simulink model "chap7_2sim_matlabfunction"  (Simulink 8.4)
settings: Solver=ode1  StartTime=0.0  StopTime=10  FixedStep=0.001  RelTol=1e-3
values from neighbouring files (symbols this model uses):
  input = [0 0.00314157198278 0.00628301994168 0.0094242198577 0.0125650477217 0.0157053795391 0.018845091335 0.0219840591589 0.0251221590899 0.028259267241 0.0313952597647 0.0345300128572 ... (10001 elements, 10001x1)]    [input.mat]
  PlantADen = [1 PlantAPara.a1 PlantAPara.a0]    [main.m]
  PlantANum = [PlantAPara.b1 PlantAPara.b0]    [main.m]
  s = u(1)    [chap7_2ctrl.m]    (also in fsmcctrl.m)
  Ts = 0.001    [main.m]
libraries: simulink x5, fod x3
settings Model: Creator=Administrator  LastModifiedBy=Administrator  ExtModeTrigMode=oneshot  ExtModeArmWhenConnect=off
settings DataIOCC: LimitDataPoints=off  SignalLoggingName=sigsOut
settings OptimizationCC: BooleanDataType=off  ExpressionDepthLimit=128
settings DebuggingCC: SaveWithParameterizedLinksMsg=none  SignalResolutionControl=TryResolveAllWithWarning  SolverPrmCheckMsg=none  MultiTaskDSMMsg=warning  MultiTaskCondExecSysMsg=none  FcnCallInpInsideContextMsg=EnableAllAsError  StateNameClashWarn=none
settings HardwareCC: TargetLongLongMode=on  TargetIntDivRoundTo=Zero  TargetEndianess=LittleEndian  TargetHWDeviceType=MATLAB Host  ProdEqTarget=off
settings RTWCC: IncludeERTFirstTime=on

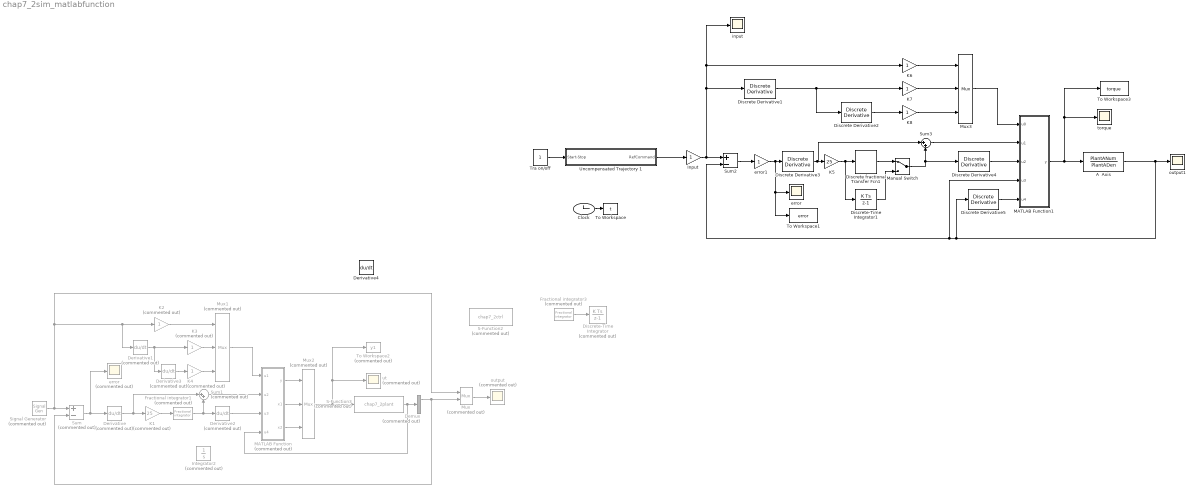
== system chap7_2sim_matlabfunction ==
  A  Axis : DiscreteTransferFcn  Numerator=PlantANum  Denominator=PlantADen  SampleTime=Ts
  Clock : Clock
  Demux : Demux  Commented=on  Outputs=2
  Derivative{,1..3} (4 alike) : Derivative  Commented=on
  Derivative4 : Derivative
  Discrete Derivative{1..5} (5 alike) : simulink/Discrete/Discrete Derivative  gainval=1.0  ICPrevScaledInput=0.0  InputProcessing=Inherited  OutMin=[]  OutMax=[]  OutDataType=fixdt(1, 16)  OutScaling=2^-10  DoSatur=off
  Discrete fractional Transfer Fcn1 : fod/Discrete fractional Transfer Fcn  zeroPoly=1  polePoly=s^0.9  freqRange=[0.001, 1000]  approxNum=5  useRef=off  dscrMethod=Matched  wc=0  ts=0.001
  Discrete-Time Integrator : DiscreteIntegrator  Commented=on  InitialConditionSetting=State (most efficient)
  Discrete-Time Integrator1 : DiscreteIntegrator  InitialConditionSetting=State (most efficient)  SampleTime=0.001
  Fractional integrator1 : fod/Fractional integrator  Commented=on  gam=0.7  ww=[0.001; 1000]  n=3  nFod=off
  Fractional integrator3 : fod/Fractional integrator  Commented=on  gam=0.9  ww=[0.001; 1000]  n=3  nFod=off
  Input : Gain  SampleTime=0.001
  Integrator2 : Integrator  Commented=on
  K1 : Gain  Commented=on  Gain=25
  K2 : Gain  Commented=on
  K3 : Gain  Commented=on
  K4 : Gain  Commented=on
  K5 : Gain  Gain=25  SampleTime=0.001
  K6 : Gain
  K7 : Gain
  K8 : Gain
  MATLAB Function : MATLAB Function  Commented=on  TreatAsAtomicUnit=on
  MATLAB Function1 : MATLAB Function  TreatAsAtomicUnit=on
  Manual Switch : ManualSwitch
  Mux : Mux  Commented=on  Inputs=2
  Mux1 : Mux  Commented=on  Inputs=3
  Mux2 : Mux  Commented=on  Inputs=3
  Mux3 : Mux  Inputs=3
  S-Function2 : S-Function  Commented=on  FunctionName=chap7_2ctrl  EnableBusSupport=off
  S-Function3 : S-Function  Commented=on  FunctionName=chap7_2plant  EnableBusSupport=off
  Signal Generator : SignalGenerator  Commented=on
  Sum : Sum  Commented=on  Inputs=+-  SaturateOnIntegerOverflow=on  InputSameDT=on  OutDataTypeStr=Inherit: Same as first input
  Sum1 : Sum  Commented=on  Inputs=|++
  Sum2 : Sum  Inputs=+-  SampleTime=0.001  SaturateOnIntegerOverflow=on  InputSameDT=on  OutDataTypeStr=Inherit: Same as first input
  Sum3 : Sum  Inputs=|++  SampleTime=0.001
  To Workspace : ToWorkspace  VariableName=t  SampleTime=-1
  To Workspace1 : ToWorkspace  VariableName=error  SampleTime=-1
  To Workspace2 : ToWorkspace  Commented=on  VariableName=y1  SampleTime=-1
  To Workspace3 : ToWorkspace  VariableName=torque  SampleTime=-1
  "Tra on/off " : Constant  SampleTime=0.001
  Uncompensated Trajectory 1 : Subsystem
  error : Scope  Commented=on
      settings: SaveName=ScopeData2
  "error " : Scope
      settings: SaveName=ScopeData5
  error1 : Gain  SampleTime=0.001
  "input " : Scope
      settings: SaveName=ScopeData4
  output : Scope  Commented=on
  output1 : Scope
  "torque " : Scope
      settings: SaveName=ScopeData6
  ut : Scope  Commented=on
      settings: SaveName=ScopeData3
  wires:
  Clock/1 -> To Workspace/1
  Mux2/1 -> To Workspace2/1, ut/1, S-Function3/1
  Mux/1 -> output/1
  Sum/1 -> Derivative/1, error/1
  Signal Generator/1 -> K2/1, Derivative1/1, Mux/1, Sum/1
  Demux/1 -> Sum/2, Mux/2
  Derivative/1 -> Sum1/1, K1/1
  Sum1/1 -> MATLAB Function/2(u2)
  K1/1 -> Fractional integrator1/1
  Fractional integrator1/1 -> Derivative2/1, Sum1/2
  Derivative2/1 -> MATLAB Function/3(u3)
  Derivative1/1 -> K3/1, Derivative3/1
  Derivative3/1 -> K4/1
  K2/1 -> Mux1/1
  K3/1 -> Mux1/2
  K4/1 -> Mux1/3
  Mux1/1 -> MATLAB Function/1(u1)
  S-Function3/1 -> MATLAB Function/4(u4), Demux/1
  MATLAB Function/1(y) -> Mux2/1
  MATLAB Function/2(x1) -> Mux2/2
  MATLAB Function/3(x2) -> Mux2/3
  Sum2/1 -> error1/1
  Discrete Derivative3/1 -> Sum3/1, K5/1
  Sum3/1 -> MATLAB Function1/2(u1)
  K5/1 -> Discrete-Time Integrator1/1, Discrete fractional Transfer Fcn1/1
  Discrete fractional Transfer Fcn1/1 -> Manual Switch/1
  Discrete Derivative4/1 -> MATLAB Function1/3(u2)
  A  Axis/1 -> Discrete Derivative5/1, Sum2/2, MATLAB Function1/4(u3), output1/1
  Discrete Derivative5/1 -> MATLAB Function1/5(u4)
  "Tra on/off "/1 -> Uncompensated Trajectory 1/1(Start-Stop)
  error1/1 -> To Workspace1/1, "error "/1, Discrete Derivative3/1
  Discrete Derivative1/1 -> Discrete Derivative2/1, K7/1
  Discrete Derivative2/1 -> K8/1
  K6/1 -> Mux3/1
  K7/1 -> Mux3/2
  K8/1 -> Mux3/3
  Mux3/1 -> MATLAB Function1/1(u0)
  Input/1 -> Discrete Derivative1/1, "input "/1, K6/1, Sum2/1
  MATLAB Function1/1(y) -> To Workspace3/1, "torque "/1, A  Axis/1
  Fractional integrator3/1 -> Discrete-Time Integrator/1
  Uncompensated Trajectory 1/1(RefCommand) -> Input/1
  Discrete-Time Integrator1/1 -> Manual Switch/2
  Manual Switch/1 -> Discrete Derivative4/1, Sum3/2

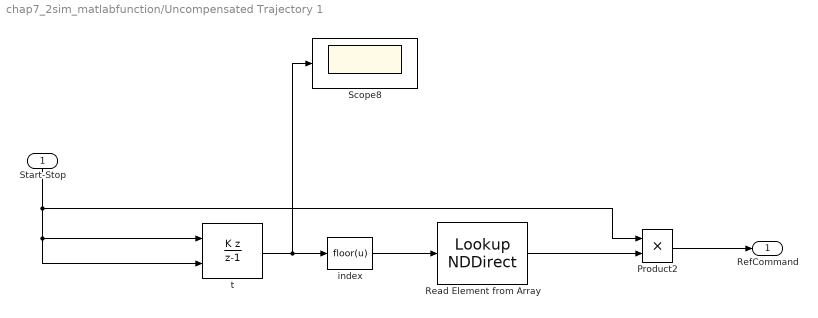
== system chap7_2sim_matlabfunction/Uncompensated Trajectory 1 ==
  Start-Stop : Inport
  Product2 : Product  RndMeth=Zero
  Read Element from Array : LookupNDDirect  NumberOfTableDimensions=1  Table=input
  Scope8 : Scope
      settings: YMin=-50  YMax=250  SaveName=ScopeData9
  index : Fcn  Expr=floor(u)
  t : DiscreteIntegrator  IntegratorMethod=Accumulation: Backward Euler  ExternalReset=rising  SampleTime=Ts
  RefCommand : Outport
  wires:
  Read Element from Array/1 -> Product2/2
  t/1 -> Scope8/1, index/1
  Product2/1 -> RefCommand/1
  Start-Stop/1 -> Product2/1, t/1, t/2
  index/1 -> Read Element from Array/1

== matlab function MATLAB Function1 ==
  data: u0 input double; u1 input double; y output double; u2 input double; u3 input double; u4 input double
function y= fcn(u0,u1,u2,u3,u4)
%#codegen

%t=0:0.001:10;

%r=0.5*sin(2*pi*t);
%dr=0.5*2*pi*cos(2*pi*t);
%ddr=-0.5*(2*pi)^2*sin(2*pi*t);

r=u0(1);
dr=u0(2);
ddr=u0(3);

s=u1;
fde=u2;
%q、dq
x1=u3;
x2=u4;

m=0.1101;
c=0.4001;

if x2>0
    dt=0.11847;
else
    dt=-0.11466;
end

k1=5;
k2=0.5;
%k1=5;
%k2=0.5;

ut=m*(ddr+fde+k1*s+k2*sign(s))+c*x2+dt;

y = ut;

== matlab function MATLAB Function ==
  data: u1 input double; y output double; u2 input double; u3 input double; u4 input double; x1 output double; x2 output double
function [y,x1,x2]= fcn(u1,u2,u3,u4)
%#codegen

%t=0:0.001:10;

%r=0.5*sin(2*pi*t);
%dr=0.5*2*pi*cos(2*pi*t);
%ddr=-0.5*(2*pi)^2*sin(2*pi*t);

r=u1(1);
dr=u1(2);
ddr=u1(3);

s=u2;
fde=u3;
%q、dq
x1=u4(1);
x2=u4(2);

m=0.2146;
c=1.994;

if x2>0
    dt=0.8788;
else
    dt=-0.94645;
end

k1=5;
k2=0.5;
%k1=5;
%k2=0.5;

ut=m*(ddr+fde+k1*s+k2*sign(s))+c*x2+dt;

y = ut;
